simulink model "bai2"  (R2017b)
settings: Solver=ode5  StartTime=0.0  StopTime=1200  FixedStep=0.05  RelTol=1e-3
undefined symbols (not defined in the file or in its folder): sigbuilder_block
libraries: fuzblock x1
settings Model: Creator=phamt  LastModifiedBy=phamt

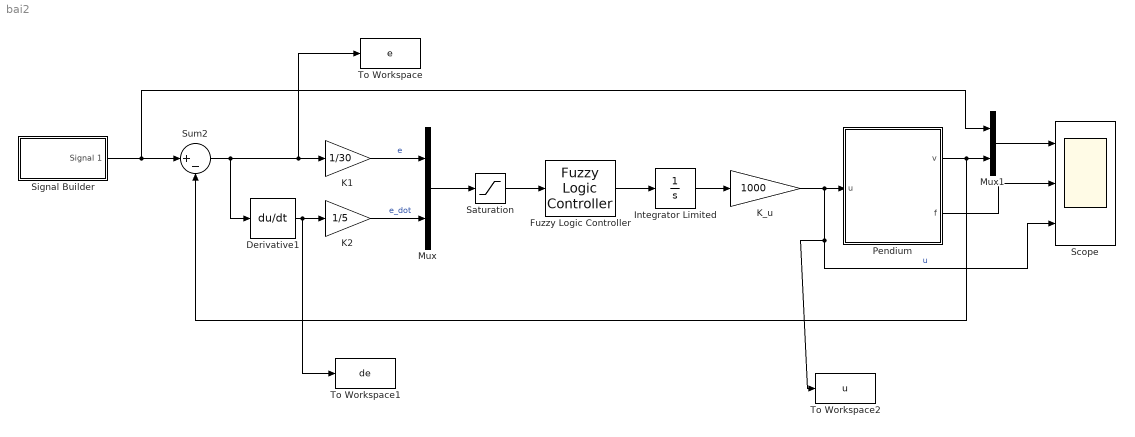
== system bai2 ==
  Derivative1 : Derivative
  Fuzzy Logic Controller : fuzblock/Fuzzy Logic  Controller  FIS='bai2_PI_FIS.fis'  OutputSampleNumber=101  DataType=double  FuzzifiedInputs=off  RuleFiringStrengths=off  RuleOutputs=off  AggregatedOutputs=off  SimulateUsing=Interpreted execution
  Integrator Limited : Integrator  LimitOutput=on  UpperSaturationLimit=1  LowerSaturationLimit=-1
  K1 : Gain  Gain=1/30
  K2 : Gain  Gain=1/5
  K_u : Gain  Gain=1000
  Mux : Mux  Inputs=2
  Mux1 : Mux  Inputs=2
  Pendium : Subsystem  mask{m=1300, Ap=0.3, d=100, t=0.2, v0=0, f0=0}
  Saturation : Saturate  UpperLimit=1  LowerLimit=-1
  Scope : Scope  NumInputPorts=3
  Signal Builder : Subsystem  Tag=STV Subsys  LoadFcn=sigbuilder_block('load',[0 36 960 449.5 ]);  StartFcn=sigbuilder_block('start');  StopFcn=sigbuilder_block('stop');  ClipboardFcn=sigbuilder_block('clipboard');  mask(Sigbuilder block){tuvar=[0:10]}
      mask help: Simulink:masks:SigbuilderBlock_MD
      mask init:
      | if ~strcmp(get_param(bdroot(gcbh),'SimulationStatus'),'stopped') tuvar = sigbuilder_block('maskInit'); end
      settings: CopyFcn=sigbuilder_block('copy');  DeleteFcn=sigbuilder_block('delete');  ModelCloseFcn=sigbuilder_block('modelClose');  PreSaveFcn=sigbuilder_block('preSave');  PauseFcn=sigbuilder_block('pause');  ContinueFcn=sigbuilder_block('continue');  NameChangeFcn=sigbuilder_block('namechange');  OpenFcn=sigbuilder_block('open',[437.6 199.2 550.4 400 ]);  CloseFcn=sigbuilder_block('close');
      mask Display: plot(0, 0, 100, 100,[2, 2, 32, 32, 2], [68, 8, 8, 68, 68],[32, 2], [38, 38], [32, 19, 2],[53, 60, 44], [32, 17, 17, 2],[16, 16, 31, 31]);txt = getActiveGroup(gcbh);text(2, 100, txt,'verticalAlignment', 'top');
  Sum2 : Sum  Inputs=|+-
  To Workspace : ToWorkspace  VariableName=e  SampleTime=-1
  To Workspace1 : ToWorkspace  VariableName=de  SampleTime=-1
  To Workspace2 : ToWorkspace  VariableName=u  SampleTime=-1
  wires:
  Signal Builder/1(Signal 1) -> Mux1/1, Sum2/1
  Derivative1/1 -> To Workspace1/1, K2/1
  Mux/1 -> Saturation/1
  K2/1 -> Mux/2  "e_dot"
  Sum2/1 -> Derivative1/1, To Workspace/1, K1/1
  Fuzzy Logic Controller/1 -> Integrator Limited/1
  K1/1 -> Mux/1  "e"
  Saturation/1 -> Fuzzy Logic Controller/1
  Mux1/1 -> Scope/1
  Integrator Limited/1 -> K_u/1
  Pendium/1(v) -> Sum2/2, Mux1/2
  K_u/1 -> To Workspace2/1, Scope/3, Pendium/1(u)  "u"
  Pendium/2(f) -> Scope/2

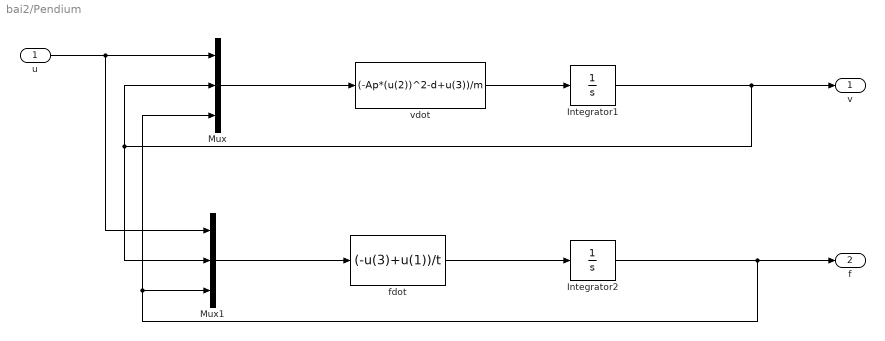
== system bai2/Pendium ==
  u : Inport
  Integrator1 : Integrator  InitialCondition=v0
  Integrator2 : Integrator  InitialCondition=f0
  Mux : Mux  Inputs=3
  Mux1 : Mux  Inputs=3
  fdot : Fcn  Expr=(-u(3)+u(1))/t
  vdot : Fcn  Expr=(-Ap*(u(2))^2-d+u(3))/m
  v : Outport
  f : Outport  Port=2
  wires:
  Integrator2/1 -> Mux1/3, Mux/3, f/1
  Integrator1/1 -> Mux1/2, Mux/2, v/1
  vdot/1 -> Integrator1/1
  fdot/1 -> Integrator2/1
  u/1 -> Mux1/1, Mux/1
  Mux1/1 -> fdot/1
  Mux/1 -> vdot/1

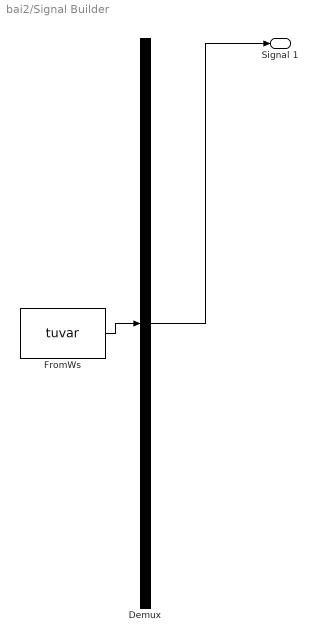
== system bai2/Signal Builder ==
  Demux : Demux  Tag=STV Demux  Outputs=1
  FromWs : FromWorkspace  Tag=STV FromWs  VariableName=tuvar  SampleTime=0
      SigBuilderData=|
      | common.afterFinalStr = 'Extrapolate'
      | common.sampleTime = 0
      | dataSet.timeRange = [0 1200]
      | dataSet.name = 'Group 1'
      | sbobj.Groups.Name = 'Group 1'
      | sbobj.Groups.Signals.Name = 'Signal 1'
      | sbobj.Groups.Signals.XData = [0 200 200 400 400 600 600 800 800 1000 1000 1200]
      | sbobj.Groups.Signals.YData = [30 30 20 20 10 10 25 25 15 15 30 30]
      | sbobj.Groups.TimeRange = [0 1200]
  Signal 1 : Outport  Tag=STV Outport
  wires:
  Demux/1 -> Signal 1/1
  FromWs/1 -> Demux/1
